simulink library "components_lib"  (Simulink 6.2)
undefined symbols (not defined in the file): A_ang_c, A_att_c, A_est, A_kalman, albedo_onboard_wrapper, B_ang_c, B_att_c, B_est, B_kalman, C_ang_c, C_att_c, C_est, C_i, C_kalman, C_p, Cd, D_ang_c, D_att_c, D_est, D_kalman, Dim, DiscIntNeverNeededParam, Hr, Hs, inerti, Ki, Kr, Ks, magnitude, otoquest, otoquest_with_pro, qmethod, rho, sat_temp_start, ss_proj3, sun_emu_angles2currents, sun_emu_vec2angles, Ts, vector_projection_onto_plane, w_mw_i, w_mw_init, zenith2ref
libraries: components_lib x163, simulink x44, albedo_lib x4, Accessories_lib x3, simulink_extras x2, discrete_bdot_filter x1
(part 3 of 5)

== system components_lib/ADS/On-board model/Albedo emulation model ==
  Sunlight vector(I) : Inport  Port=1  LatchInput=off
  Nadir vector (I) : Inport  Port=2  LatchInput=off
  q(I>E) : Inport  Port=3  LatchInput=off
  Earth Albedo Model1 : albedo_lib/Earth Albedo Model  eprdata=mean_epr  redfac=1  Ts=60  enable=on
  Vector rotation by q1 : components_lib/Math utilities/Vector operations/Vector rotation by q
  Vector rotation by q2 : components_lib/Math utilities/Vector operations/Vector rotation by q
  Reflectivity matrix : Outport
  wires:
  Vector rotation by q1/1 -> Earth Albedo Model1/1
  Vector rotation by q2/1 -> Earth Albedo Model1/2
  Earth Albedo Model1/1 -> Reflectivity matrix/1
  Nadir vector (I)/1 -> Vector rotation by q1/2
  q(I>E)/1 -> Vector rotation by q1/1, Vector rotation by q2/1
  Sunlight vector(I)/1 -> Vector rotation by q2/2

== system components_lib/ADS/On-board model/Albedo model onboard ==
  "Earth -> Sun vector (ECEF)" : Inport  Port=1  LatchInput=off
  Zenith vector (ECEF) : Inport  Port=2  LatchInput=off
  q(I->S) : Inport  Port=3  LatchInput=off
  q(I->E) : Inport  Port=4  LatchInput=off
  On : Constant  Orientation=down  Value=enable
  On1 : Constant  Orientation=down  Value=~enable
  Sum : Sum  Inputs=|++
  cos dependent albedo : Subsystem
  fov matrix albedo : Subsystem
  Albedo vector (I) : Outport
  wires:
  On1/1 -> cos dependent albedo/Enable
  fov matrix albedo/1(Albedo vector (I)) -> Sum/2
  cos dependent albedo/1(Albedo vector (I)) -> Sum/1
  On/1 -> fov matrix albedo/Enable
  Zenith vector (ECEF)/1 -> fov matrix albedo/1(Zenith vector (ECEF)), cos dependent albedo/2(Zenith vector (ECEF))
  "Earth -> Sun vector (ECEF)"/1 -> fov matrix albedo/2("Earth -> Sun vector (ECEF)"), cos dependent albedo/1("Earth -> Sun vector (ECEF)")
  q(I->E)/1 -> fov matrix albedo/4(q(I->E))
  q(I->S)/1 -> fov matrix albedo/3(q(I->S))
  Sum/1 -> Albedo vector (I)/1

== system components_lib/ADS/On-board model/Albedo projection ==
  Reflectivity matrix : Inport  Port=1  LatchInput=off
  Nadir (E) : Inport  Port=2  LatchInput=off
  q(S->E) : Inport  Port=3  LatchInput=off
  Mux7 : Mux
  Reshape : simulink/Math Operations/Reshape  OutputDimensionality=1-D array  OutputDimensions=[1,1]
  Vector rotation by q : components_lib/Math utilities/Quaternion operations/Vector rotation by q
  Vector rotation by q1 : components_lib/Math utilities/Quaternion operations/Vector rotation by q
  X+ vector (SC) : Constant  Value=[1 0 0]
  ss_proj : MATLABFcn  MATLABFcn=ss_proj3(u(length(u)-8:length(u)-6),u(length(u)-5:length(u)-3),u(length(u)-2:length(u)),reshape(u(1:length(u)-9),round([180,288]/sqrt(51840/(length(u)-9)))))
  y+ vector (SC) : Constant  Value=[0 1 0]
  Albedo flux [W/m^2] : Outport
  wires:
  ss_proj/1 -> Albedo flux [W/m^2]/1
  Mux7/1 -> ss_proj/1
  Reshape/1 -> Mux7/1
  Vector rotation by q/1 -> Mux7/3
  Vector rotation by q1/1 -> Mux7/4
  y+ vector (SC)/1 -> Vector rotation by q1/2
  X+ vector (SC)/1 -> Vector rotation by q/2
  q(S->E)/1 -> Vector rotation by q1/1, Vector rotation by q/1
  Nadir (E)/1 -> Mux7/2  "nadir"
  Reflectivity matrix/1 -> Reshape/1

== system components_lib/ADS/On-board model/Eclipse model ==
  note: theta_e
  Sun vector (I) : Inport  Port=1  LatchInput=off
  Satellite (I) : Inport  Port=2  LatchInput=off
  Constant : Constant  Value=pi
  Divide : Product  Inputs=*/  OutScaling=2^-10
  Dot Product : simulink/Math Operations/Dot Product  InputSameDT=on  OutDataType=sfix(16)  OutScaling=2^-10  DoSatur=off
  Dot Product1 : simulink/Math Operations/Dot Product  InputSameDT=on  OutDataType=sfix(16)  OutScaling=2^-10  DoSatur=off
  Earth radius : Constant  Value=r_e
  False : Constant  Value=0
  Manual Switch : simulink/Signal Routing/Manual Switch  sw=0  action=0
  Math Function : Math  Operator=sqrt  SaturateOnIntegerOverflow=on
  Max angle : Constant  Value=theta_e/180*pi
  Satellite unit vector : components_lib/Math utilities/Vector operations/to unit vector
  Sum : Sum  Orientation=down  Inputs=-+|
  Sum1 : Sum  Inputs=+-|
  Sun unit vector : components_lib/Math utilities/Vector operations/to unit vector
  Switch : Switch
  Trigonometric Function : Trigonometry  Operator=asin
  Trigonometric Function1 : Trigonometry  Operator=acos
  True : Constant
  "Eclipse: 1 = true, 0 = false" : Outport  PortDimensions=1
  wires:
  Dot Product1/1 -> Math Function/1
  Max angle/1 -> Manual Switch/1
  Trigonometric Function/1 -> Manual Switch/2
  Manual Switch/1 -> Sum1/2
  Switch/1 -> "Eclipse: 1 = true, 0 = false"/1
  False/1 -> Switch/1
  True/1 -> Switch/3
  Sum1/1 -> Switch/2
  Sum/1 -> Sum1/1  "theta"
  Constant/1 -> Sum/2
  Trigonometric Function1/1 -> Sum/1
  Divide/1 -> Trigonometric Function/1
  Math Function/1 -> Divide/2
  Earth radius/1 -> Divide/1
  Dot Product/1 -> Trigonometric Function1/1
  Satellite unit vector/1 -> Dot Product/2
  Sun unit vector/1 -> Dot Product/1
  Satellite (I)/1 -> Dot Product1/2, Dot Product1/1, Satellite unit vector/1
  Sun vector (I)/1 -> Sun unit vector/1

== system components_lib/ADS/On-board model/Ephemeris on-board ==
  Time t(JD) : Inport  Port=1  LatchInput=off
  ECEF : Subsystem
  Sun Position : Subsystem
  Earth Rotation q(I->E) : Outport
  Sun Position R_s(I) : Outport  Port=2
  wires:
  ECEF/1(q(I->E)) -> Earth Rotation q(I->E)/1  "q(I -> E)"
  Time t(JD)/1 -> Sun Position/1(t(JD)), ECEF/1(t(JD))  "t"
  Sun Position/1(R_s(I)) -> Sun Position R_s(I)/1  "R_s(I)"

== system components_lib/ADS/On-board model/Gyros ==
  Temperature_meas [K] : Inport  Port=1  LatchInput=off
  V_ADC [mV] : Inport  Port=2  LatchInput=off
  Combine the angular rate  from the 6 gyros to angular  rate in S-frame : Subsystem
  Compensate op.amp gain1 : Gain  Gain=1./op_amp_gain
  Compensate op.amp gain2 : Gain  Gain=1./op_amp_gain
  Divide : Product  Inputs=*/  OutScaling=2^-10
  Drift(offset) [mV/K] : Constant  Value=e_drift_offset_obc_alg
  Drift(scale factor) [%/K] : Constant  Value=e_drift_scale_obc_alg
  Gain : Gain  Gain=0.01
  Offset [mV] : Constant  Value=offset_obc_alg
  Produc3 : Product  Inputs=3  SaturateOnIntegerOverflow=on
  Product : Product  RndMeth=Zero
  Product1 : Product  SaturateOnIntegerOverflow=on
  Sign : Signum  Orientation=down
  Sum1 : Sum  Inputs=|+-
  Sum2 : Sum  Inputs=|++
  Sum3 : Sum  Inputs=+-
  Sum4 : Sum  Inputs=+-
  "mV->rad/s " : Constant  Value=scale_obc_alg
  temp must be deviation  from 25 degree C : Constant  Orientation=up  Value=298.15
  W_meas (S) meaned pair [rad/s] : Outport
  W_meas (S) [rad/s] : Outport  Port=2
  wires:
  Combine the angular rate  from the 6 gyros to angular  rate in S-frame/1(W_meas (S)) -> W_meas (S) meaned pair [rad/s]/1
  Compensate op.amp gain1/1 -> Sum3/2
  Compensate op.amp gain2/1 -> Sum3/1
  Sum2/1 -> Divide/2  "Scale factor"
  Produc3/1 -> Sum2/1  "temp coor"
  "mV->rad/s "/1 -> Produc3/3, Sum2/2
  Gain/1 -> Produc3/2
  Temperature_meas [K]/1 -> Sum1/1
  temp must be deviation  from 25 degree C/1 -> Sum1/2
  Drift(offset) [mV/K]/1 -> Product1/1
  Divide/1 -> Combine the angular rate  from the 6 gyros to angular  rate in S-frame/1(W_meas 6 gyros), W_meas (S) [rad/s]/1
  Sum1/1 -> Product1/2, Produc3/1
  Offset [mV]/1 -> Compensate op.amp gain1/1
  V_ADC [mV]/1 -> Compensate op.amp gain2/1
  Drift(scale factor) [%/K]/1 -> Gain/1
  Product1/1 -> Product/2
  Sign/1 -> Product/1
  Sum3/1 -> Sign/1, Sum4/1
  Product/1 -> Sum4/2
  Sum4/1 -> Divide/1

== system components_lib/ADS/On-board model/Magnetic field model ==
  R_sc(E) : Inport  Port=1  LatchInput=off
  S-Function : S-Function  FunctionName=igrfS  Parameters=2002,4
  B(E) : Outport
  wires:
  S-Function/1 -> B(E)/1
  R_sc(E)/1 -> S-Function/1

== system components_lib/ADS/On-board model/Magnetometer ==
  V_ADC [mV] : Inport  Port=1  LatchInput=off
  temp_meas [K] : Inport  Port=2  LatchInput=off
  Compensate  op.amp gain2 : Gain  Gain=1./op_amp_gain
  Divide : Product  Inputs=*/  OutScaling=2^-10
  Drift(scale factor) [%/K] : Constant  Value=e_drift_sens_obc_alg
  Offset [mV] : Constant  Orientation=up  Value=op_amp_offset
  Product3 : Product  Inputs=3  SaturateOnIntegerOverflow=on
  Sum1 : Sum  Inputs=-+|
  Sum2 : Sum  Inputs=|++
  Sum3 : Sum  Inputs=|+-
  convert ppm to scale factor : Gain  Gain=10e-6
  mv/v/gauss-> mv/gauss : Gain  Gain=v_supply_model
  sensitivity  [mV/V/Gauss] : Constant  Value=sens_obc_alg
  temp must be deviation  from 25 degree C : Constant  Orientation=down  Value=298.15
  Mag field meas [Gauss] : Outport
  wires:
  Divide/1 -> Mag field meas [Gauss]/1
  temp must be deviation  from 25 degree C/1 -> Sum1/1
  temp_meas [K]/1 -> Sum1/2
  mv/v/gauss-> mv/gauss/1 -> Divide/2  "Scale factor"
  Compensate  op.amp gain2/1 -> Divide/1
  Sum3/1 -> Compensate  op.amp gain2/1
  Drift(scale factor) [%/K]/1 -> convert ppm to scale factor/1
  V_ADC [mV]/1 -> Sum3/1
  Offset [mV]/1 -> Sum3/2
  Sum1/1 -> Product3/1
  convert ppm to scale factor/1 -> Product3/2
  sensitivity  [mV/V/Gauss]/1 -> Sum2/2, Product3/3
  Product3/1 -> Sum2/1  "temp coor"
  Sum2/1 -> mv/v/gauss-> mv/gauss/1

== system components_lib/ADS/On-board model/Orbit and Magnetic field models ==
  note: Other TLE
  note: Ørsted TLE
  JD : Inport  Port=1  LatchInput=off
  Earth rotation q(I->E) : Inport  Port=2  LatchInput=off
  " S-Function" : S-Function  FunctionName=sgp4S
  Constant : Constant  Value=enable_oersted_tle
  Constant1 : Constant  Value=enable_other_tle
  Demux1 : Demux  Outputs=[3 3]
  Gain 1440 : Gain  Orientation=down  Gain=1440  SaturateOnIntegerOverflow=on
  Magnetic field model : components_lib/ADS/On-board model/Magnetic field model
  Mux : Mux  Inputs=2
  Quaternion inverter : components_lib/Math utilities/Quaternion operations/Quaternion inverter
  Sum : Sum  Orientation=down  Inputs=-+|  SaturateOnIntegerOverflow=on  InputSameDT=on
  Sum1 : Sum  SaturateOnIntegerOverflow=on  InputSameDT=on
  Sum2 : Sum  SaturateOnIntegerOverflow=on  InputSameDT=on
  T->Gauss : Gain  Gain=1e4  SaturateOnIntegerOverflow=on
  TLE and time initialization1 : Subsystem  mask{satname='Orsted', YYDDD=02039, JulianDay=2452275.5+40.69255057, xndt2o=0.00002748*0, xndd6o=0, bstar=0.00071190, xincl=96.4788, xnodeo=112.1945, eo=0.0148615, omegao=71.6037, xmo=290.1241, xno=14.43891950, ts=1}
      mask prompts: satname "Satellite Name:"; YYDDD "Epoch [YYDDD]:"; JulianDay "Epoch [JD]:"; xndt2o "MM dot:"; xndd6o "MM dot dot:"; bstar "Drag:"; xincl "Inclination [deg]:"; xnodeo "Right Ascension of Ascending Node [deg]:"; eo "Eccentricity [-]:"; omegao "Argument of Perigee [deg]:"; xmo "Mean Anomaly [deg]:"; xno "Mean Motion [rev/day]:"; ts "Sampling Time [sec]:"
      mask help:
      | Input TLE from the standard Two-Line Orbital Element Set Format
      | Satellite Name, Line 1 and 2.
  TLE and time initialization3 : Subsystem  mask{satname='Orsted', YYDDD=02039, JulianDay=2452275.5+40.69255057, xndt2o=0.00002748*0, xndd6o=0, bstar=0.00071190, xincl=96.4788, xnodeo=112.1945, eo=0.0148615, omegao=71.6037, xmo=290.1241, xno=14.43891950, ts=1}
      mask prompts: satname "Satellite Name:"; YYDDD "Epoch [YYDDD]:"; JulianDay "Epoch [JD]:"; xndt2o "MM dot:"; xndd6o "MM dot dot:"; bstar "Drag:"; xincl "Inclination [deg]:"; xnodeo "Right Ascension of Ascending Node [deg]:"; eo "Eccentricity [-]:"; omegao "Argument of Perigee [deg]:"; xmo "Mean Anomaly [deg]:"; xno "Mean Motion [rev/day]:"; ts "Sampling Time [sec]:"
      mask help:
      | Input TLE from the standard Two-Line Orbital Element Set Format
      | Satellite Name, Line 1 and 2.
  Terminator : Terminator
  Vector rotation by q : components_lib/Math utilities/Vector operations/Vector rotation by q
  Vector rotation by q1 : components_lib/Math utilities/Vector operations/Vector rotation by q
  "km -> m" : Gain  Gain=1000  SaturateOnIntegerOverflow=on
  "km/s -> m/s" : Gain  Gain=1000  SaturateOnIntegerOverflow=on
  Magnetic field vector B(I) : Outport
  Position (I) : Outport  Port=2
  wires:
  T->Gauss/1 -> Magnetic field vector B(I)/1
  Vector rotation by q1/1 -> T->Gauss/1
  Quaternion inverter/1 -> Vector rotation by q1/1
  Magnetic field model/1 -> Vector rotation by q1/2  "B(I / E)"
  Earth rotation q(I->E)/1 -> Quaternion inverter/1, Vector rotation by q/1
  Vector rotation by q/1 -> Magnetic field model/1
  Sum1/1 -> Mux/2
  Gain 1440/1 -> Mux/1
  Sum/1 -> Gain 1440/1
  Sum2/1 -> Sum/1
  Demux1/1 -> "km -> m"/1
  Demux1/2 -> "km/s -> m/s"/1
  " S-Function"/1 -> Demux1/1
  Mux/1 -> " S-Function"/1
  "km/s -> m/s"/1 -> Terminator/1
  "km -> m"/1 -> Position (I)/1, Vector rotation by q/2
  JD/1 -> Sum/2
  Constant1/1 -> TLE and time initialization3/1(Enable?)
  Constant/1 -> TLE and time initialization1/1(Enable?)
  TLE and time initialization1/1(Oersted_InitJD) -> Sum2/1
  TLE and time initialization3/1(Other_InitJD) -> Sum2/2
  TLE and time initialization1/2(Oersted_TLE) -> Sum1/1
  TLE and time initialization3/2(Other_TLE) -> Sum1/2

== system components_lib/ADS/On-board model/Sun sensors ==
  note: Vector plus sides minus
      | vector minus sides
  I_ADC [mA] : Inport  Port=1  LatchInput=off
  Temperature  [K] : Inport  Port=2  LatchInput=off
  Compensate op_amp gain (is an attenuation) : Gain  Gain=op_amp_gain
  Demux : Demux  Outputs=2
  Drift [%/degreesC] : Constant  Value=temp_drift
  Max currents : Constant  Value=I_max
  Normalization of currents : Product  Inputs=*/  OutScaling=2^-10
  Normalized darkcurrents : Constant  Value=I_dark./I_max
  Offset [mV] : Constant  Orientation=up  Value=op_amp_offset
  Sum1 : Sum  Inputs=|+-  SaturateOnIntegerOverflow=on
  Sum2 : Sum  Inputs=|+-
  Sum3 : Sum  Inputs=|+-
  Sum5 : Sum  Inputs=|+-
  Sum6 : Sum  Inputs=++|  SaturateOnIntegerOverflow=on
  Temp is deviation from 25 degree C : Constant  Orientation=up  Value=298.15
  Temperature  drift [mA] : Product  Inputs=3  SaturateOnIntegerOverflow=on
  Sun position (s) : Outport
  wires:
  Temp is deviation from 25 degree C/1 -> Sum5/2
  Sum5/1 -> Temperature  drift [mA]/3
  Temperature  [K]/1 -> Sum5/1
  Drift [%/degreesC]/1 -> Temperature  drift [mA]/2
  Temperature  drift [mA]/1 -> Sum6/2
  Demux/1 -> Sum1/1
  Demux/2 -> Sum1/2
  Sum1/1 -> Sun position (s)/1
  Normalized darkcurrents/1 -> Sum2/2
  Sum2/1 -> Demux/1
  Compensate op_amp gain (is an attenuation)/1 -> Temperature  drift [mA]/1, Sum6/1
  Max currents/1 -> Normalization of currents/2
  Normalization of currents/1 -> Sum2/1
  Sum6/1 -> Normalization of currents/1
  I_ADC [mA]/1 -> Sum3/1
  Offset [mV]/1 -> Sum3/2
  Sum3/1 -> Compensate op_amp gain (is an attenuation)/1

== system components_lib/ADS/On-board model/Temperature: Convert voltage from ADC into measured temperature ==
  Temperature_meas [mV] : Inport  Port=1  LatchInput=off
  Temperature [K] : Outport
  wires:
  Temperature_meas [mV]/1 -> Temperature [K]/1

== system components_lib/ADS/On-board model/sensor model ==
  Magnetometer V_ADC [mV] : Inport  Port=1  LatchInput=off
  Gyros V_ADC [mV] : Inport  Port=2  LatchInput=off
  Sun sensors [mA] : Inport  Port=3  LatchInput=off
  Temperature V_ADC [mV] : Inport  Port=4  LatchInput=off
  Gyros : components_lib/ADS/On-board model/Gyros  op_amp_gain=[10 10 10 10 10 10]  op_amp_offset=[2500 2500 2500 2500 2500 2500]  scale_obc_alg=[859.4 859.4 859.4 859.4 859.4 859.4 ]  offset_obc_alg=[2500 2500 2500 2500 2500 2500]  e_drift_scale_obc_alg=[0.075 0.075 0.075 0.075 0.075 0.075]  e_drift_offset_obc_alg=[10 10 10 10 10 10]
  Mag field vector  to unit vector : components_lib/Math utilities/Vector operations/to unit vector
  Magnetometer : components_lib/ADS/On-board model/Magnetometer  op_amp_gain=[500 500 500]  v_supply_model=5  op_amp_offset=[2500 2500 2500]  sens_obc_alg=[1 1 1]  e_drift_sens_obc_alg=[-3000 -3000 -3000]  e_offset_obc_alg=[10 10 10]*0
  Sun pos vector  to unit vector : components_lib/Math utilities/Vector operations/to unit vector
  Sun sensors : components_lib/ADS/On-board model/Sun sensors  op_amp_gain=1  op_amp_offset=0  temp_drift=0.00233  I_dark=[0.0815 0.0815 0.0815 0.0815 0.0815 0.0815 ]  I_max=[1.3928 1.3928 1.3928 1.3928 1.3928 1.3928]
  Temperature: Convert voltage from ADC into measured temperature : components_lib/ADS/On-board model/Temperature: Convert voltage from ADC into measured temperature
  Magnetic field unit vector (S) : Outport
  Sun unit vector (S) : Outport  Port=2
  Omega (1x3) (S) [rad/s] : Outport  Port=3
  Omega (1x6) (S) [rad/s] : Outport  Port=4
  wires:
  Sun pos vector  to unit vector/1 -> Sun unit vector (S)/1
  Gyros/2 -> Omega (1x6) (S) [rad/s]/1
  Mag field vector  to unit vector/1 -> Magnetic field unit vector (S)/1
  Sun sensors/1 -> Sun pos vector  to unit vector/1
  Sun sensors [mA]/1 -> Sun sensors/1
  Gyros V_ADC [mV]/1 -> Gyros/2
  Gyros/1 -> Omega (1x3) (S) [rad/s]/1
  Temperature V_ADC [mV]/1 -> Temperature: Convert voltage from ADC into measured temperature/1
  Magnetometer/1 -> Mag field vector  to unit vector/1
  Magnetometer V_ADC [mV]/1 -> Magnetometer/1
  Temperature: Convert voltage from ADC into measured temperature/1 -> Sun sensors/2, Magnetometer/2, Gyros/1

== system components_lib/Actuator Emulation/Magnetorquer/electro mechanics transfer function ==
  v : Inport  Port=1  LatchInput=off
  R(T) : Inport  Port=2  LatchInput=off
  Integrator : Integrator
  Product1 : Product  RndMeth=Zero
  Sum : Sum  Inputs=|+-
  dot Gain : Gain  Gain=1/L_mt
  i : Outport
  wires:
  R(T)/1 -> Product1/1
  v/1 -> Sum/1
  Product1/1 -> Sum/2
  Integrator/1 -> i/1, Product1/2
  dot Gain/1 -> Integrator/1
  Sum/1 -> dot Gain/1

== system components_lib/Actuator Emulation/Momentum wheel/Mechanical TF ==
  N_mw : Inport  Port=1  LatchInput=off
  Constant : Constant  Value=mu_f
  Gain : Gain  Gain=1/I_mw
  Integrator : Integrator  InitialCondition=w_mw_init
  Product : Product  RndMeth=Zero
  Sum : Sum  Inputs=|+-
  w_mw : Outport
  wires:
  Gain/1 -> Integrator/1
  Sum/1 -> Gain/1
  Product/1 -> Sum/2
  N_mw/1 -> Sum/1
  Constant/1 -> Product/1
  Integrator/1 -> Product/2, w_mw/1

== system components_lib/Disturbances/Exposed area/Projection Matrix1 ==
  n-vector : Inport  Port=1  LatchInput=off
  Add : Sum  Inputs=+++  OutScaling=2^-10
  Demux : Demux  Outputs=3
  Gain{1..6} (6 alike) : Gain  Gain=-1
  Math Funcion : Math  Operator=square  SaturateOnIntegerOverflow=on
  Math Function : Math  Operator=reciprocal  SaturateOnIntegerOverflow=on
  Math Function1 : Math  Operator=square  SaturateOnIntegerOverflow=on
  Math Function2 : Math  Operator=square  SaturateOnIntegerOverflow=on
  Mux : Mux  Inputs=9
  Product1 : Product  RndMeth=Zero
  Product2 : Product  RndMeth=Zero
  Product3 : Product  RndMeth=Zero
  Prouct : Product  RndMeth=Zero
  Reshape : simulink/Math Operations/Reshape  OutputDimensionality=Customize  OutputDimensions=[3,3]
  Sum : Sum  Inputs=|++
  Sum1 : Sum  Inputs=+|+
  Sum2 : Sum  Inputs=++|
  P matrix : Outport
  wires:
  Demux/1 -> Math Funcion/1, Product1/1, Product2/1
  Demux/2 -> Math Function1/1, Product1/2, Product3/1
  Demux/3 -> Product2/2, Math Function2/1, Product3/2
  Gain1/1 -> Mux/2
  Gain2/1 -> Mux/3
  Gain3/1 -> Mux/4
  Gain4/1 -> Mux/6
  Gain5/1 -> Mux/7
  Gain6/1 -> Mux/8
  Product1/1 -> Gain1/1, Gain3/1
  Product2/1 -> Gain2/1, Gain5/1
  Product3/1 -> Gain4/1, Gain6/1
  Sum/1 -> Mux/1
  Sum2/1 -> Mux/9
  Sum1/1 -> Mux/5
  Math Funcion/1 -> Sum1/1, Sum2/1, Add/1
  Math Function2/1 -> Sum1/2, Sum/2, Add/3
  Math Function1/1 -> Sum2/2, Sum/1, Add/2
  Mux/1 -> Reshape/1
  n-vector/1 -> Demux/1
  Math Function/1 -> Prouct/1
  Add/1 -> Math Function/1
  Reshape/1 -> Prouct/2
  Prouct/1 -> P matrix/1

== system components_lib/Disturbances/Exposed area/Satellite Area ==
  px : Inport  Port=1  LatchInput=off
  py : Inport  Port=2  LatchInput=off
  pz : Inport  Port=3  LatchInput=off
  Dot Product : simulink/Math Operations/Dot Product  InputSameDT=on  OutDataType=sfix(16)  OutScaling=2^-10  DoSatur=off
  Dot Product1 : simulink/Math Operations/Dot Product  InputSameDT=on  OutDataType=sfix(16)  OutScaling=2^-10  DoSatur=off
  Dot Product2 : simulink/Math Operations/Dot Product  InputSameDT=on  OutDataType=sfix(16)  OutScaling=2^-10  DoSatur=off
  Sum : Sum  Inputs=+|+|+
  cross_product_no_fnc1 : components_lib/Math utilities/Vector operations/cross_product_no_fnc
  cross_product_no_fnc2 : components_lib/Math utilities/Vector operations/cross_product_no_fnc
  cross_product_no_fnc3 : components_lib/Math utilities/Vector operations/cross_product_no_fnc
  inv1 : Math  Operator=sqrt  SaturateOnIntegerOverflow=on
  inv2 : Math  Operator=sqrt  SaturateOnIntegerOverflow=on
  inv3 : Math  Operator=sqrt  SaturateOnIntegerOverflow=on
  area_sat : Outport
  wires:
  Sum/1 -> area_sat/1
  inv3/1 -> Sum/3
  inv2/1 -> Sum/2
  pz/1 -> cross_product_no_fnc2/2, cross_product_no_fnc1/2
  cross_product_no_fnc2/1 -> Dot Product2/1, Dot Product2/2
  Dot Product2/1 -> inv3/1
  cross_product_no_fnc1/1 -> Dot Product1/2, Dot Product1/1
  Dot Product1/1 -> inv2/1
  py/1 -> cross_product_no_fnc2/1, cross_product_no_fnc3/2
  inv1/1 -> Sum/1
  px/1 -> cross_product_no_fnc1/1, cross_product_no_fnc3/1
  cross_product_no_fnc3/1 -> Dot Product/1, Dot Product/2
  Dot Product/1 -> inv1/1

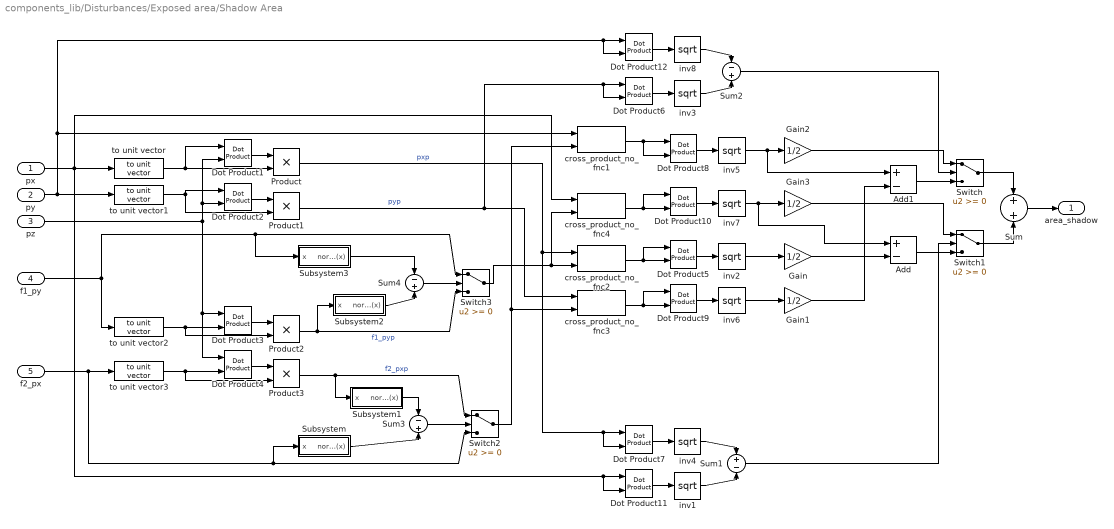
== system components_lib/Disturbances/Exposed area/Shadow Area ==
  px : Inport  Port=1  LatchInput=off
  py : Inport  Port=2  LatchInput=off
  pz : Inport  Port=3  LatchInput=off
  f1_py : Inport  Port=4  LatchInput=off
  f2_px : Inport  Port=5  LatchInput=off
  Add : Sum  Inputs=+-  OutScaling=2^-10
  Add1 : Sum  Inputs=+-  OutScaling=2^-10
  Dot Product{1..12} (12 alike) : simulink/Math Operations/Dot Product  InputSameDT=on  OutDataType=sfix(16)  OutScaling=2^-10  DoSatur=off
  Gain{,1..3} (4 alike) : Gain  Gain=1/2
  Product{,1..3} (4 alike) : Product  RndMeth=Zero
  Subsystem : Subsystem
  Subsystem1 : Subsystem
  Subsystem2 : Subsystem
  Subsystem3 : Subsystem
  Sum : Sum  Inputs=+|+
  Sum1 : Sum  Inputs=+|-
  Sum2 : Sum  Inputs=-|+
  Sum3 : Sum  Inputs=-|+
  Sum4 : Sum  Inputs=-|+
  Switch{,1..3} (4 alike) : Switch
  cross_product_no_fnc{1..4} (4 alike) : components_lib/Math utilities/Vector operations/cross_product_no_fnc  Tag=cross_product_no_fnc
  inv{1..8} (8 alike) : Math  Operator=sqrt  SaturateOnIntegerOverflow=on
  to unit vector{,1..3} (4 alike) : components_lib/Math utilities/Vector operations/to unit vector
  area_shadow : Outport
  wires:
  Subsystem1/1(norm(x)) -> Sum3/1
  Subsystem2/1(norm(x)) -> Sum4/2
  Subsystem3/1(norm(x)) -> Sum4/1
  Subsystem/1(norm(x)) -> Sum3/2
  Sum4/1 -> Switch3/2
  Switch3/1 -> cross_product_no_fnc4/2, cross_product_no_fnc2/2
  Sum3/1 -> Switch2/2
  Product3/1 -> Switch2/1, Subsystem1/1(x)  "f2_pxp"
  inv8/1 -> Sum2/1
  inv3/1 -> Sum2/2
  inv1/1 -> Sum1/2
  inv4/1 -> Sum1/1
  Sum1/1 -> Switch1/2
  Sum2/1 -> Switch/2
  Dot Product12/1 -> inv8/1
  Dot Product11/1 -> inv1/1
  Dot Product1/1 -> Product/1
  Dot Product2/1 -> Product1/1
  Dot Product3/1 -> Product2/1
  Dot Product4/1 -> Product3/1
  Switch1/1 -> Sum/2
  Switch/1 -> Sum/1
  Gain3/1 -> Switch1/1
  Add/1 -> Switch1/3
  Gain2/1 -> Switch/1
  Add1/1 -> Switch/3
  Gain1/1 -> Add1/2
  Gain/1 -> Add/2
  inv7/1 -> Add/1, Gain3/1
  inv5/1 -> Gain2/1, Add1/1
  inv6/1 -> Gain1/1
  inv2/1 -> Gain/1
  Product1/1 -> Dot Product6/2, Dot Product6/1, cross_product_no_fnc3/1  "pyp"
  Product2/1 -> Subsystem2/1(x), Switch3/3  "f1_pyp"
  Dot Product10/1 -> inv7/1
  cross_product_no_fnc4/1 -> Dot Product10/1, Dot Product10/2
  Dot Product9/1 -> inv6/1
  cross_product_no_fnc3/1 -> Dot Product9/1, Dot Product9/2
  Dot Product5/1 -> inv2/1
  cross_product_no_fnc2/1 -> Dot Product5/1, Dot Product5/2
  Dot Product8/1 -> inv5/1
  cross_product_no_fnc1/1 -> Dot Product8/1, Dot Product8/2
  Dot Product7/1 -> inv4/1
  Switch2/1 -> cross_product_no_fnc1/2, cross_product_no_fnc3/2
  Dot Product6/1 -> inv3/1
  Product/1 -> cross_product_no_fnc2/1, Dot Product7/2, Dot Product7/1  "pxp"
  Sum/1 -> area_shadow/1
  pz/1 -> Dot Product2/2, Dot Product1/2, Dot Product4/1, Dot Product3/1
  to unit vector1/1 -> Product1/2, Dot Product2/1
  to unit vector2/1 -> Product2/2, Dot Product3/2
  to unit vector3/1 -> Product3/2, Dot Product4/2
  to unit vector/1 -> Product/2, Dot Product1/1
  f2_px/1 -> Switch2/3, Subsystem/1(x), to unit vector3/1
  f1_py/1 -> Subsystem3/1(x), Switch3/1, to unit vector2/1
  py/1 -> Dot Product12/2, Dot Product12/1, cross_product_no_fnc1/1, to unit vector1/1
  px/1 -> Dot Product11/2, Dot Product11/1, cross_product_no_fnc4/1, to unit vector/1

== system components_lib/Disturbances/Exposed area/Solar Array Area ==
  f1_py : Inport  Port=1  LatchInput=off
  px : Inport  Port=2  LatchInput=off
  py : Inport  Port=3  LatchInput=off
  f2_px : Inport  Port=4  LatchInput=off
  Dot Product : simulink/Math Operations/Dot Product  InputSameDT=on  OutDataType=sfix(16)  OutScaling=2^-10  DoSatur=off
  Dot Product1 : simulink/Math Operations/Dot Product  InputSameDT=on  OutDataType=sfix(16)  OutScaling=2^-10  DoSatur=off
  Gain : Gain  Gain=2
  Gain1 : Gain  Gain=2
  Sum1 : Sum  Inputs=+|||+
  cross_product_no_fnc1 : components_lib/Math utilities/Vector operations/cross_product_no_fnc
  cross_product_no_fnc3 : components_lib/Math utilities/Vector operations/cross_product_no_fnc
  inv1 : Math  Operator=sqrt  SaturateOnIntegerOverflow=on
  inv2 : Math  Operator=sqrt  SaturateOnIntegerOverflow=on
  area_flaps : Outport
  wires:
  Sum1/1 -> area_flaps/1
  Gain1/1 -> Sum1/2
  inv2/1 -> Gain1/1
  Dot Product1/1 -> inv2/1
  cross_product_no_fnc1/1 -> Dot Product1/2, Dot Product1/1
  py/1 -> cross_product_no_fnc1/1
  px/1 -> cross_product_no_fnc3/2
  f2_px/1 -> cross_product_no_fnc1/2
  Gain/1 -> Sum1/1
  inv1/1 -> Gain/1
  Dot Product/1 -> inv1/1
  cross_product_no_fnc3/1 -> Dot Product/2, Dot Product/1
  f1_py/1 -> cross_product_no_fnc3/1

== system components_lib/Disturbances/Gravity/Gravity Gradient Torque ==
  note: To principal frame
  R_sc(I) : Inport  Port=1  LatchInput=off
  I(C) : Inport  Port=2  LatchInput=off
  q(C->S) : Inport  Port=3  LatchInput=off
  q(I->S) : Inport  Port=4  LatchInput=off
  " " : Subsystem
  3*GM : Gain  Gain=3*G*M_earth  SaturateOnIntegerOverflow=on
  Constant : Constant  Value=3
  Constant1 : Constant  Value=[1 0 0;0 1 0;0 0 1]
  Constant2 : Constant  Value=[1 1 1]  VectorParams1D=off
  Dot roduct : simulink/Math Operations/Dot Product  InputSameDT=on  OutDataType=sfix(16)  OutScaling=2^-10  DoSatur=off
  Product : Product  Multiplication=Matrix(*)  SaturateOnIntegerOverflow=on
  Product1 : Product  SaturateOnIntegerOverflow=on
  Product2 : Product  Multiplication=Matrix(*)  SaturateOnIntegerOverflow=on
  Product3 : Product  SaturateOnIntegerOverflow=on
  R : Math  Operator=pow  SaturateOnIntegerOverflow=on
  Vector rotation by q : components_lib/Math utilities/Vector operations/Vector rotation by q
  cross_product_no_fnc : components_lib/Math utilities/Vector operations/cross_product_no_fnc
  inv : Math  Operator=reciprocal  SaturateOnIntegerOverflow=on
  inv1 : Math  Operator=sqrt  SaturateOnIntegerOverflow=on
  to unit vector : components_lib/Math utilities/Vector operations/to unit vector
  N_gr(S) : Outport
  wires:
  Vector rotation by q/1 -> Product3/2
  3*GM/1 -> Product3/1
  R_sc(I)/1 -> " "/3(R_sc(I)), Dot roduct/1, Dot roduct/2
  Constant1/1 -> Product1/2
  Product2/1 -> Product1/1
  Constant2/1 -> Product2/2
  I(C)/1 -> Product2/1
  Product/1 -> cross_product_no_fnc/2
  Product1/1 -> Product/1
  " "/1(R_sc(C)) -> to unit vector/1
  q(I->S)/1 -> " "/2("q(I -> SC)")
  q(C->S)/1 -> " "/1(q(C->SC)), Vector rotation by q/1
  to unit vector/1 -> Product/2, cross_product_no_fnc/1
  Constant/1 -> R/2
  inv1/1 -> inv/1
  inv/1 -> R/1
  R/1 -> 3*GM/1
  Product3/1 -> N_gr(S)/1
  Dot roduct/1 -> inv1/1
  cross_product_no_fnc/1 -> Vector rotation by q/2

== system components_lib/Disturbances/Gravity/Gravity Moon ==
  R_m_sat(I) : Inport  Port=1  LatchInput=off
  M_sat : Inport  Port=2  LatchInput=off
  G*M_m : Constant  Value=G*M_moon
  Gain : Gain  Gain=-1  SaturateOnIntegerOverflow=on
  Math Function1 : Math  Operator=reciprocal  SaturateOnIntegerOverflow=on
  Math Function2 : Math  Operator=magnitude^2  SaturateOnIntegerOverflow=on
  Product : Product  SaturateOnIntegerOverflow=on
  Product1 : Product  SaturateOnIntegerOverflow=on
  Product2 : Product  SaturateOnIntegerOverflow=on
  to unit vector1 : components_lib/Math utilities/Vector operations/to unit vector
  F_m(I) : Outport
  wires:
  Product/1 -> Product2/2
  Gain/1 -> Product2/1
  Product2/1 -> F_m(I)/1
  to unit vector1/1 -> Gain/1
  Product1/1 -> Product/2
  Math Function1/1 -> Product/1
  G*M_m/1 -> Product1/2
  M_sat/1 -> Product1/1
  Math Function2/1 -> Math Function1/1
  R_m_sat(I)/1 -> to unit vector1/1, Math Function2/1

== system components_lib/Disturbances/Gravity/Gravity Sun ==
  M_sat : Inport  Port=1  LatchInput=off
  R_s_sat(I) : Inport  Port=2  LatchInput=off
  G*M_s : Constant  Value=G*M_sun
  Gain : Gain  Gain=-1  SaturateOnIntegerOverflow=on
  Math Function1 : Math  Operator=reciprocal  SaturateOnIntegerOverflow=on
  Math Function2 : Math  Operator=magnitude^2  SaturateOnIntegerOverflow=on
  Product : Product  SaturateOnIntegerOverflow=on
  Product1 : Product  SaturateOnIntegerOverflow=on
  Product2 : Product  SaturateOnIntegerOverflow=on
  to unit vector : components_lib/Math utilities/Vector operations/to unit vector
  F_s(I) : Outport
  wires:
  Product/1 -> Product2/2
  Gain/1 -> Product2/1
  R_s_sat(I)/1 -> to unit vector/1, Math Function2/1
  Product2/1 -> F_s(I)/1
  to unit vector/1 -> Gain/1
  Product1/1 -> Product/2
  Math Function1/1 -> Product/1
  G*M_s/1 -> Product1/2
  M_sat/1 -> Product1/1
  Math Function2/1 -> Math Function1/1

== system components_lib/Disturbances/Gravity/Zonal Harmonics  Earth ==
  R_sat(I) : Inport  Port=1  LatchInput=off
  Cartesian to Spherical : simulink_extras/Transformations/Cartesian to Spherical
  Demux : Demux  Outputs=3
  Demux1 : Demux  Outputs=3
  Mux : Mux  Inputs=3
  Mux1 : Mux  Inputs=3
  S-Function : S-Function  FunctionName=zonal
  Spherical to Cartesian : simulink_extras/Transformations/Spherical to Cartesian
  Terminator : Terminator
  grad(U_zonal(I)) : Outport
  wires:
  Demux/2 -> Terminator/1
  R_sat(I)/1 -> Demux1/1
  Spherical to Cartesian/2 -> Mux/2
  Cartesian to Spherical/2 -> Spherical to Cartesian/2, Mux1/2
  Cartesian to Spherical/3 -> Mux1/3
  Cartesian to Spherical/1 -> Mux1/1
  Mux1/1 -> S-Function/1
  S-Function/1 -> Demux/1
  Demux/3 -> Spherical to Cartesian/3
  Demux/1 -> Spherical to Cartesian/1
  Spherical to Cartesian/3 -> Mux/3
  Spherical to Cartesian/1 -> Mux/1
  Mux/1 -> grad(U_zonal(I))/1
  Demux1/3 -> Cartesian to Spherical/3
  Demux1/2 -> Cartesian to Spherical/2
  Demux1/1 -> Cartesian to Spherical/1

== system components_lib/Disturbances/Magnetic residual disturbance/Magnetic field E->S ==
  q(I->S) : Inport  Port=1  LatchInput=off
  q(I->E) : Inport  Port=2  LatchInput=off
  B(E) : Inport  Port=3  LatchInput=off
  Quaternion inverter : Accessories_lib/Math utilities/Quaternion operations/Quaternion inverter
  Vector rotation by q : Accessories_lib/Math utilities/Vector operations/Vector rotation by q
  Vector rotation by q1 : Accessories_lib/Math utilities/Vector operations/Vector rotation by q
  B(S) : Outport
  wires:
  Quaternion inverter/1 -> Vector rotation by q/1
  Vector rotation by q/1 -> Vector rotation by q1/2
  q(I->S)/1 -> Vector rotation by q1/1
  Vector rotation by q1/1 -> B(S)/1
  q(I->E)/1 -> Quaternion inverter/1
  B(E)/1 -> Vector rotation by q/2

== system components_lib/Math utilities/Quaternion operations/Quarternion error ==
  note: 
  q : Inport  Port=1  LatchInput=off
  q2 : Inport  Port=2  LatchInput=off
  Quaternion inverter1 : components_lib/Math utilities/Quaternion operations/Quaternion inverter
  qmul no func : components_lib/Math utilities/Quaternion operations/qmul no func
  "\"q1-q2\"" : Outport
  wires:
  Quaternion inverter1/1 -> qmul no func/1
  q2/1 -> qmul no func/2
  q/1 -> Quaternion inverter1/1
  qmul no func/1 -> "\"q1-q2\""/1

== system components_lib/Math utilities/Quaternion operations/Quaternion inverter ==
  q : Inport  Port=1  LatchInput=off
  Demux : Demux
  Demux1 : Demux  Outputs=3
  Gain : Gain  Gain=-1  SaturateOnIntegerOverflow=on
  Mux : Mux
  Mux1 : Mux  Inputs=3
  q^-1 : Outport
  wires:
  q/1 -> Demux/1
  Mux/1 -> q^-1/1
  Demux/4 -> Mux/4
  Demux/1 -> Mux1/1
  Demux/2 -> Mux1/2
  Demux/3 -> Mux1/3
  Mux1/1 -> Gain/1
  Demux1/1 -> Mux/1
  Demux1/2 -> Mux/2
  Demux1/3 -> Mux/3
  Gain/1 -> Demux1/1

== system components_lib/Math utilities/Quaternion operations/Reverse quaternion rotation ==
  q : Inport  Port=1  LatchInput=off
  Quaternion inverter : Subsystem
  q_opposit : Outport
  wires:
  q/1 -> Quaternion inverter/1(q)
  Quaternion inverter/1(q^-1) -> q_opposit/1

== system components_lib/Math utilities/Quaternion operations/Rotation from q1 to q2 ==
  q1 : Inport  Port=1  LatchInput=off
  q2 : Inport  Port=2  LatchInput=off
  Quaternion inverter : components_lib/Math utilities/Quaternion operations/Quaternion inverter
  Quaternion mulitiplication : S-Function  FunctionName=qmul
  q_diff : Outport
  wires:
  q2/1 -> Quaternion inverter/1
  Quaternion inverter/1 -> Quaternion mulitiplication/2
  Quaternion mulitiplication/1 -> q_diff/1
  q1/1 -> Quaternion mulitiplication/1

== system components_lib/Math utilities/Quaternion operations/Rotation of q1 by q2 ==
  q1 : Inport  Port=1  LatchInput=off
  q2 : Inport  Port=2  LatchInput=off
  Quaternion mulitiplication : S-Function  FunctionName=qmul
  q_res : Outport
  wires:
  q1/1 -> Quaternion mulitiplication/1
  q2/1 -> Quaternion mulitiplication/2
  Quaternion mulitiplication/1 -> q_res/1

== system components_lib/Math utilities/Quaternion operations/Vector rotation by q ==
  q : Inport  Port=1  LatchInput=off
  V : Inport  Port=2  LatchInput=off
  Constant : Constant  Value=0
  Demux : Demux  Outputs=3
  Demux1 : Demux
  Mux : Mux
  Mux1 : Mux  Inputs=3
  Quaternion inverter : Subsystem
  Terminator : Terminator
  qmul no func : components_lib/Math utilities/Quaternion operations/qmul no func
  qmul no func1 : components_lib/Math utilities/Quaternion operations/qmul no func
  q'Vq : Outport
  wires:
  qmul no func/1 -> qmul no func1/2
  Quaternion inverter/1(q^-1) -> qmul no func1/1
  Mux/1 -> qmul no func/1
  q/1 -> qmul no func/2, Quaternion inverter/1(q)
  V/1 -> Demux/1
  Demux/1 -> Mux/1
  Demux/2 -> Mux/2
  Demux/3 -> Mux/3
  Constant/1 -> Mux/4
  qmul no func1/1 -> Demux1/1
  Demux1/1 -> Mux1/1
  Demux1/2 -> Mux1/2
  Demux1/3 -> Mux1/3
  Demux1/4 -> Terminator/1
  Mux1/1 -> q'Vq/1

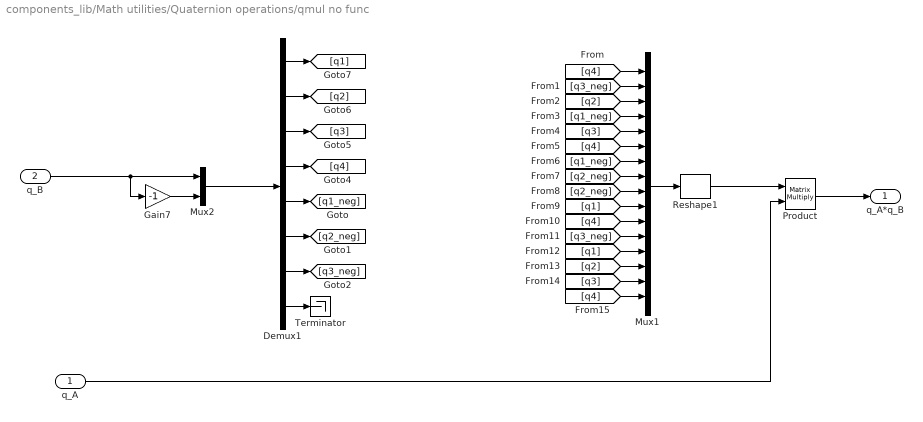
== system components_lib/Math utilities/Quaternion operations/qmul no func ==
  q_A : Inport  Port=1  LatchInput=off
  q_B : Inport  Port=2  LatchInput=off
  Demux1 : Demux  Outputs=8
  Gain7 : Gain  Gain=-1
  Mux1 : Mux  Inputs=16
  Mux2 : Mux  Inputs=2
  Product : Product  Multiplication=Matrix(*)  RndMeth=Zero
  Reshape1 : simulink/Math Operations/Reshape  OutputDimensionality=Customize  OutputDimensions=[4,4]
  Terminator : Terminator
  q_A*q_B : Outport
  wires:
  Product/1 -> q_A*q_B/1
  q_A/1 -> Product/2
  q_B/1 -> Gain7/1, Mux2/1
  [q4] -> Mux1/16
  [q3] -> Mux1/15
  [q2] -> Mux1/14
  [q1] -> Mux1/13
  [q3_neg] -> Mux1/12
  [q4] -> Mux1/11
  [q1] -> Mux1/10
  [q2_neg] -> Mux1/9
  [q2_neg] -> Mux1/8
  [q1_neg] -> Mux1/7
  [q4] -> Mux1/6
  [q3] -> Mux1/5
  [q1_neg] -> Mux1/4
  [q2] -> Mux1/3
  [q3_neg] -> Mux1/2
  [q4] -> Mux1/1
  Demux1/8 -> Terminator/1
  Demux1/7 -> [q3_neg]
  Demux1/6 -> [q2_neg]
  Demux1/5 -> [q1_neg]
  Demux1/4 -> [q4]
  Demux1/3 -> [q3]
  Demux1/2 -> [q2]
  Demux1/1 -> [q1]
  Gain7/1 -> Mux2/2
  Mux1/1 -> Reshape1/1
  Mux2/1 -> Demux1/1
  Reshape1/1 -> Product/1

== system components_lib/Math utilities/Quaternion operations/quaternion composition ==
  vector : Inport  Port=1  LatchInput=off
  angle : Inport  Port=2  LatchInput=off
  Demux : Demux  Outputs=3
  Gain : Gain  Gain=1/2  SaturateOnIntegerOverflow=on
  Mux : Mux
  Product : Product  SaturateOnIntegerOverflow=on
  Trigonometric Function : Trigonometry  Operator=cos
  Trigonometric Function1 : Trigonometry
  to unit vector : components_lib/Math utilities/Vector operations/to unit vector
  q : Outport
  wires:
  angle/1 -> Gain/1
  Gain/1 -> Trigonometric Function/1, Trigonometric Function1/1
  vector/1 -> to unit vector/1
  to unit vector/1 -> Product/1
  Trigonometric Function1/1 -> Product/2
  Product/1 -> Demux/1
  Demux/1 -> Mux/1
  Demux/2 -> Mux/2
  Demux/3 -> Mux/3
  Trigonometric Function/1 -> Mux/4
  Mux/1 -> q/1

== system components_lib/Math utilities/Quaternion operations/quaternion decomposition ==
  q_in : Inport  Port=1  LatchInput=off
  Demux : Demux
  Gain : Gain  Gain=2  SaturateOnIntegerOverflow=on
  Math Function : Math  Operator=reciprocal  SaturateOnIntegerOverflow=on
  Mux : Mux  Inputs=3
  Product : Product  SaturateOnIntegerOverflow=on
  Trigonometric Function : Trigonometry  Operator=acos
  Trigonometric Function1 : Trigonometry
  to unit vector : components_lib/Math utilities/Vector operations/to unit vector
  Vector : Outport
  Angle : Outport  Port=2
  wires:
  q_in/1 -> Demux/1
  Demux/4 -> Trigonometric Function/1
  Trigonometric Function/1 -> Gain/1, Trigonometric Function1/1
  Gain/1 -> Angle/1
  Demux/1 -> Mux/1
  Demux/2 -> Mux/2
  Demux/3 -> Mux/3
  Mux/1 -> Product/1
  Math Function/1 -> Product/2
  Trigonometric Function1/1 -> Math Function/1
  Product/1 -> to unit vector/1
  to unit vector/1 -> Vector/1

== system components_lib/Math utilities/Quaternion operations/quaternion expansion ==
  q1-3 : Inport  Port=1  LatchInput=off
  Constant1 : Constant
  Demux2 : Demux  Outputs=3
  Math Function4 : Math  Operator=square  SaturateOnIntegerOverflow=on
  Math Function5 : Math  Operator=square  SaturateOnIntegerOverflow=on
  Math Function6 : Math  Operator=square  SaturateOnIntegerOverflow=on
  Math Function7 : Math  Operator=sqrt  SaturateOnIntegerOverflow=on
  Mux2 : Mux  Inputs=2
  Product : Product  Inputs=*/  RndMeth=Zero
  Sum1 : Sum  Inputs=++++
  q : Outport
  wires:
  Product/1 -> q/1
  Mux2/1 -> Product/1
  Math Function6/1 -> Sum1/4
  Math Function5/1 -> Sum1/3
  Math Function4/1 -> Sum1/2
  Constant1/1 -> Mux2/2, Sum1/1
  Math Function7/1 -> Product/2
  Sum1/1 -> Math Function7/1
  q1-3/1 -> Mux2/1, Demux2/1
  Demux2/3 -> Math Function6/1
  Demux2/2 -> Math Function5/1
  Demux2/1 -> Math Function4/1

== system components_lib/Math utilities/Quaternion operations/quaternion2euler ==
  quaternion : Inport  Port=1  LatchInput=off
  Mux : Mux  Inputs=3
  theta 1 : Fcn  Expr=-atan2((2*(u(2)*u(3) + u(1)*u(4))),(1-2*(u(1)*u(1) + u(2)*u(2))))
  theta 2 : Fcn  Expr=-asin(2*(u(1)*u(3)-u(2)*u(4)))
  theta 3 : Fcn  Expr=-atan2((2*(u(1)*u(2) + u(3)*u(4))),(1-2*(u(2)*u(2) + u(3)*u(3))))
  Euler angles : Outport
  wires:
  Mux/1 -> Euler angles/1
  quaternion/1 -> theta 3/1, theta 1/1, theta 2/1
  theta 3/1 -> Mux/3
  theta 2/1 -> Mux/2
  theta 1/1 -> Mux/1

== system components_lib/Math utilities/Quaternion operations/w to q ==
  Angular velocity : Inport  Port=1  LatchInput=off
  Initial quaternion : Inport  Port=2  LatchInput=off
  S-Function : S-Function  FunctionName=qestimator
  estimated quaternion : Outport
  wires:
  S-Function/1 -> estimated quaternion/1
  Initial quaternion/1 -> S-Function/1
  Angular velocity/1 -> S-Function/2

== system components_lib/Math utilities/Quaternion operations/||q|| ==
  q_in : Inport  Port=1  LatchInput=off
  quaternion composition : components_lib/Math utilities/Quaternion operations/quaternion composition
  quaternion decomposition : components_lib/Math utilities/Quaternion operations/quaternion decomposition
  q_out : Outport
  wires:
  q_in/1 -> quaternion decomposition/1
  quaternion decomposition/1 -> quaternion composition/1
  quaternion decomposition/2 -> quaternion composition/2
  quaternion composition/1 -> q_out/1

== system components_lib/Math utilities/Vector operations/Projection of a onto b ==
  a : Inport  Port=1  LatchInput=off
  b : Inport  Port=2  LatchInput=off
  Constant : Constant  Value=-2
  Dot Product : simulink/Math Operations/Dot Product  InputSameDT=on  OutDataType=sfix(16)  OutScaling=2^-10  DoSatur=off
  Math Function : Math  Operator=pow  SaturateOnIntegerOverflow=on
  Product : Product  Inputs=3  SaturateOnIntegerOverflow=on
  ||V|| : MATLABFcn  MATLABFcn=norm
  a_b : Outport
  wires:
  Product/1 -> a_b/1
  Math Function/1 -> Product/2
  Dot Product/1 -> Product/1
  ||V||/1 -> Math Function/1
  Constant/1 -> Math Function/2
  b/1 -> Product/3, ||V||/1, Dot Product/2
  a/1 -> Dot Product/1

== system components_lib/Math utilities/Vector operations/Vector rotation by q ==
  q : Inport  Port=1  LatchInput=off
  V : Inport  Port=2  LatchInput=off
  Constant : Constant  Value=0
  Demux : Demux  Outputs=3
  Demux1 : Demux
  Mux : Mux
  Mux1 : Mux  Inputs=3
  Quaternion inverter : Subsystem
  Quaternion mulitiplication : S-Function  FunctionName=qmul
  Quaternion mulitiplication1 : S-Function  FunctionName=qmul
  Terminator : Terminator
  q'Vq : Outport
  wires:
  Mux1/1 -> q'Vq/1
  Demux1/4 -> Terminator/1
  Demux1/3 -> Mux1/3
  Demux1/2 -> Mux1/2
  Demux1/1 -> Mux1/1
  Quaternion mulitiplication1/1 -> Demux1/1
  Quaternion mulitiplication/1 -> Quaternion mulitiplication1/1
  Mux/1 -> Quaternion mulitiplication/2
  Constant/1 -> Mux/4
  Demux/3 -> Mux/3
  Demux/2 -> Mux/2
  Demux/1 -> Mux/1
  V/1 -> Demux/1
  Quaternion inverter/1(q^-1) -> Quaternion mulitiplication/1
  q/1 -> Quaternion mulitiplication1/2, Quaternion inverter/1(q)

== system components_lib/Math utilities/Vector operations/cross_product ==
  u : Inport  Port=1  LatchInput=off
  v : Inport  Port=2  LatchInput=off
  S-Function : S-Function  FunctionName=s_cross_product
  y : Outport
  wires:
  S-Function/1 -> y/1
  v/1 -> S-Function/2
  u/1 -> S-Function/1

== system components_lib/Math utilities/Vector operations/cross_product_no_fnc ==
  v : Inport  Port=1  LatchInput=off
  u : Inport  Port=2  LatchInput=off
  Demux : Demux  Outputs=3
  Demux1 : Demux  Outputs=3
  Mux : Mux  Inputs=3
  Product{1..6} (6 alike) : Product  SaturateOnIntegerOverflow=on
  Sum : Sum  Inputs=-+|
  Sum1 : Sum  Inputs=-+|
  Sum2 : Sum  Inputs=-+|
  v x u : Outport
  wires:
  Mux/1 -> v x u/1
  Sum2/1 -> Mux/3
  Sum1/1 -> Mux/2
  Sum/1 -> Mux/1
  Demux1/1 -> Product6/1, Product2/1
  Demux/1 -> Product5/2, Product4/2
  Demux/2 -> Product6/2, Product1/2
  Demux1/3 -> Product4/1, Product1/1
  Demux/3 -> Product2/2, Product3/2
  Demux1/2 -> Product5/1, Product3/1
  Product5/1 -> Sum2/1
  Product6/1 -> Sum2/2
  Product2/1 -> Sum1/1
  Product4/1 -> Sum1/2
  Product1/1 -> Sum/1
  Product3/1 -> Sum/2
  u/1 -> Demux/1
  v/1 -> Demux1/1

== system components_lib/Math utilities/Vector operations/modulus ==
  u : Inport  Port=1  PortDimensions=1  LatchInput=off
  v : Inport  Port=2  PortDimensions=1  LatchInput=off
  S-Function : S-Function  FunctionName=s_modulus
  y : Outport  PortDimensions=1
  wires:
  v/1 -> S-Function/2
  S-Function/1 -> y/1
  u/1 -> S-Function/1

== system components_lib/Math utilities/Vector operations/norm ==
  u : Inport  Port=1  PortDimensions=3  LatchInput=off
  S-Function : S-Function  FunctionName=s_norm
  y : Outport  PortDimensions=1
  wires:
  u/1 -> S-Function/1
  S-Function/1 -> y/1

== system components_lib/Math utilities/Vector operations/pow ==
  u : Inport  Port=1  LatchInput=off
  v : Inport  Port=2  PortDimensions=1  LatchInput=off
  S-Function : S-Function  FunctionName=s_pow
  y : Outport
  wires:
  S-Function/1 -> y/1
  v/1 -> S-Function/2
  u/1 -> S-Function/1

== system components_lib/Math utilities/Vector operations/sign ==
  u : Inport  Port=1  LatchInput=off
  S-Function : S-Function  FunctionName=s_sign
  y : Outport
  wires:
  S-Function/1 -> y/1
  u/1 -> S-Function/1

== system components_lib/Math utilities/Vector operations/to unit vector ==
  "v  " : Inport  Port=1  LatchInput=off
  Constant : Constant
  Dot Product : simulink/Math Operations/Dot Product  InputSameDT=on  OutDataType=sfix(16)  OutScaling=2^-10  DoSatur=off
  Math Function : Math  Operator=reciprocal  SaturateOnIntegerOverflow=on
  Product : Product  SaturateOnIntegerOverflow=on
  Switch : Switch  Criteria=u2 ~= 0  SaturateOnIntegerOverflow=on
  sqrt : Math  Operator=sqrt  SaturateOnIntegerOverflow=on
  v_hat : Outport
  wires:
  Constant/1 -> Switch/3
  sqrt/1 -> Switch/1, Switch/2
  Switch/1 -> Math Function/1
  "v  "/1 -> Product/1, Dot Product/1, Dot Product/2
  Math Function/1 -> Product/2
  Product/1 -> v_hat/1
  Dot Product/1 -> sqrt/1

== system components_lib/Math utilities/Vector operations/vector projection onto plane ==
  SC veloc : Inport  Port=1  LatchInput=off
  v : Inport  Port=2  LatchInput=off
  MATLAB Fcn : MATLABFcn  MATLABFcn=vector_projection_onto_plane(u)
  Mux : Mux  Inputs=2
  v' : Outport
  wires:
  Mux/1 -> MATLAB Fcn/1
  v/1 -> Mux/2
  MATLAB Fcn/1 -> v'/1
  SC veloc/1 -> Mux/1

== system components_lib/Orbit and Ephemeris/Ephemeris/ECEF ==
  t(JD) : Inport  Port=1  LatchInput=off
  eci2ecef : MATLABFcn  MATLABFcn=eci2ecef  OutputDimensions=4
  q(I->E) : Outport
  wires:
  eci2ecef/1 -> q(I->E)/1
  t(JD)/1 -> eci2ecef/1

== system components_lib/Orbit and Ephemeris/Ephemeris/Moon Position ==
  t(JD)1 : Inport  Port=1  LatchInput=off
  Moon R in ECI : MATLABFcn  MATLABFcn=moon  OutputDimensions=3
  R_m(I) : Outport
  wires:
  t(JD)1/1 -> Moon R in ECI/1
  Moon R in ECI/1 -> R_m(I)/1

== system components_lib/Orbit and Ephemeris/Ephemeris/Sun Position ==
  t(JD) : Inport  Port=1  LatchInput=off
  Sun R in ECI : MATLABFcn  MATLABFcn=sun  OutputDimensions=3
  R_s(I) : Outport
  wires:
  t(JD)/1 -> Sun R in ECI/1
  Sun R in ECI/1 -> R_s(I)/1

== system components_lib/Orbit and Ephemeris/Orbit and Magnetic field models/Albedo ==
  Sunlight vector(I) : Inport  Port=1  LatchInput=off
  Nadir vector (I) : Inport  Port=2  LatchInput=off
  q(I>E) : Inport  Port=3  LatchInput=off
  Enable : EnablePort
  Earth Albedo Model : albedo_lib/Earth Albedo Model  eprdata=load('lib/albedo_toolbox/epr_data/2003/ga030101-031231')  redfac=1  Ts=10  enable=on
  Vector rotation by q1 : components_lib/Math utilities/Vector operations/Vector rotation by q
  Vector rotation by q2 : components_lib/Math utilities/Vector operations/Vector rotation by q
  Reflectivity matrix : Outport
  wires:
  Sunlight vector(I)/1 -> Vector rotation by q2/2
  q(I>E)/1 -> Vector rotation by q2/1, Vector rotation by q1/1
  Nadir vector (I)/1 -> Vector rotation by q1/2
  Earth Albedo Model/1 -> Reflectivity matrix/1
  Vector rotation by q2/1 -> Earth Albedo Model/2
  Vector rotation by q1/1 -> Earth Albedo Model/1

== system components_lib/Orbit and Ephemeris/Orbit and Magnetic field models/Custom time ==
  Initial time ti(JD) : Inport  Port=1  LatchInput=off
  Enable : EnablePort
  Clock : Clock
      settings: Decimation=10
  Sec2Day : Gain  Gain=1/86400  SaturateOnIntegerOverflow=on
  Sum : Sum  Inputs=|++
  Simulation time t(JD) : Outport
  wires:
  Initial time ti(JD)/1 -> Sum/1
  Sec2Day/1 -> Sum/2
  Clock/1 -> Sec2Day/1
  Sum/1 -> Simulation time t(JD)/1

== system components_lib/Orbit and Ephemeris/Orbit and Magnetic field models/Oersted Magnetic field ==
  Enable : EnablePort
  Oersted magnetic field (E) : FromWorkspace  VariableName=[oersted_data.time.sample_number oersted_data.mag.ECEFRF(:,1) oersted_data.mag.ECEFRF(:,2) oersted_data.mag.ECEFRF(:,3)]  SampleTime=1
  nT->Gauss : Gain  Gain=1e-5  SaturateOnIntegerOverflow=on
  Magnetic field vector B(E) : Outport
  wires:
  Oersted magnetic field (E)/1 -> nT->Gauss/1
  nT->Gauss/1 -> Magnetic field vector B(E)/1

== system components_lib/Orbit and Ephemeris/Orbit and Magnetic field models/Oersted position ==
  Enable : EnablePort
  Oersted Velocity (I) : FromWorkspace  VariableName=[oersted_data.time.sample_number oersted_data.vel.ECIRF(:,1) oersted_data.vel.ECIRF(:,2) oersted_data.vel.ECIRF(:,3) ]  SampleTime=1
  Oersted position (I) : FromWorkspace  VariableName=[oersted_data.time.sample_number oersted_data.pos.ECIRF(:,1) oersted_data.pos.ECIRF(:,2) oersted_data.pos.ECIRF(:,3) ]  SampleTime=1
  Position R(I) : Outport
  Velocity V(I) : Outport  Port=2
  wires:
  Oersted Velocity (I)/1 -> Velocity V(I)/1
  Oersted position (I)/1 -> Position R(I)/1

== system components_lib/Orbit and Ephemeris/Orbit and Magnetic field models/Oersted time ==
  Enable : EnablePort
  Day of Oersted-Data  (JD) : Constant  Value=2452315.5
  JD and sec. to Julian Date : Subsystem
  Seconds of Day (Orsted data) : FromWorkspace  VariableName=[oersted_data.time.sample_number oersted_data.time.second oersted_data.time.day]  SampleTime=1
  Simulation time t(JD) : Outport
  wires:
  JD and sec. to Julian Date/1(Julian Date (Day)) -> Simulation time t(JD)/1
  Day of Oersted-Data  (JD)/1 -> JD and sec. to Julian Date/2(Day as Julian Date)
  Seconds of Day (Orsted data)/1 -> JD and sec. to Julian Date/1(Second of Day)
